simulink library "ipc"  (Simulink 8.1)
settings: Solver=ode1  StartTime=0.0  StopTime=Inf  FixedStep=0.001  RelTol=1e-3
PostLoadFcn:
  | , if any(exist('dsrtsu_mdlpostloadfcn', 'file') == [2, 3, 6]), try dsrtsu_mdlpostloadfcn('Execute', bdroot); catch fprintf('Error in PostLoadFcn (dsrtsu_mdlpostloadfcn) for model "%s":\n %s\n', bdroot, lasterr); end, end,
undefined symbols (not defined in the file or in its folder): KIFO_OffsetToBumper_m, KIFO_TTCDefault_s
libraries: hcu_lib x2, ltc x1
settings Model: DSRTSU_INTERNAL_RTI_VER=450  DSRTSU_INTERNAL_RTI_TYPE=rti1401  RTICANMMDATA=struct('GeneralSetupData',struct('modelroot',['D:\ELN150201\Phase3\branches\Pedestrians complete local\AdasDragon\software\sw_development\arch\app\ifo'],'generalsettings',struct('filesettings',struct('destfolder',struct('Name','RTICANMM_FILES','Check',1),'buildfolder',struct('Name','.','Check',1),'AbsDestfolder',struct('Name',['D:\ELN150201\Phase3\branches\Pedestrians complete local\AdasDragon\software\sw_development\arch\app\ifo\RTICANMM_FILES']),'AbsBuildfolder',struct('Name',['D:\ELN150201\Phase3\branches\Pedestrians complete local\AdasDragon\software\sw_development\arch\app\ifo']))),'options',struct('addpaths',1,'rmpaths',1,'addtrcexclusion',logical(1),'cannavigator',struct('checkmonitoring',0),'show_usrtrc',0,'use_usrtrc',0),'advanced',struct('options',[1 1 1 1 1 1 1 1 1 1 1 1 1 1 1 1 1 1 1 1 1 1 1 1 1 1 1 1 1 1 1 1 1 1 1 1 1 1 1 1 1 1 1 1 1 1 1 1 1 1 1 1 1 1 1 1 1 1 1 1 1 1 1 1 1 1 1 1 1 1 1 1 1 1 1 1 1 1 1 1 1 1 1 1 1 1 1 1 1 1 1 1 1 1 1 1 1 1 1 1]),'MPSetup',{{}},'modelname','ipc','block','ipc'))  DSRTSU_INTERNAL_RTIFPGA=40  Creator=tescamilla  LastModifiedBy=AT015555

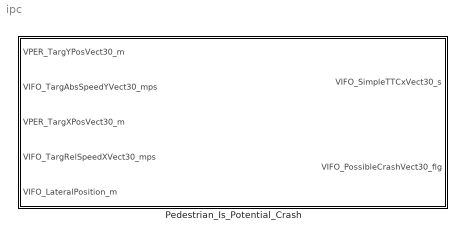
== system ipc ==
  Pedestrian_Is_Potential_Crash : Subsystem

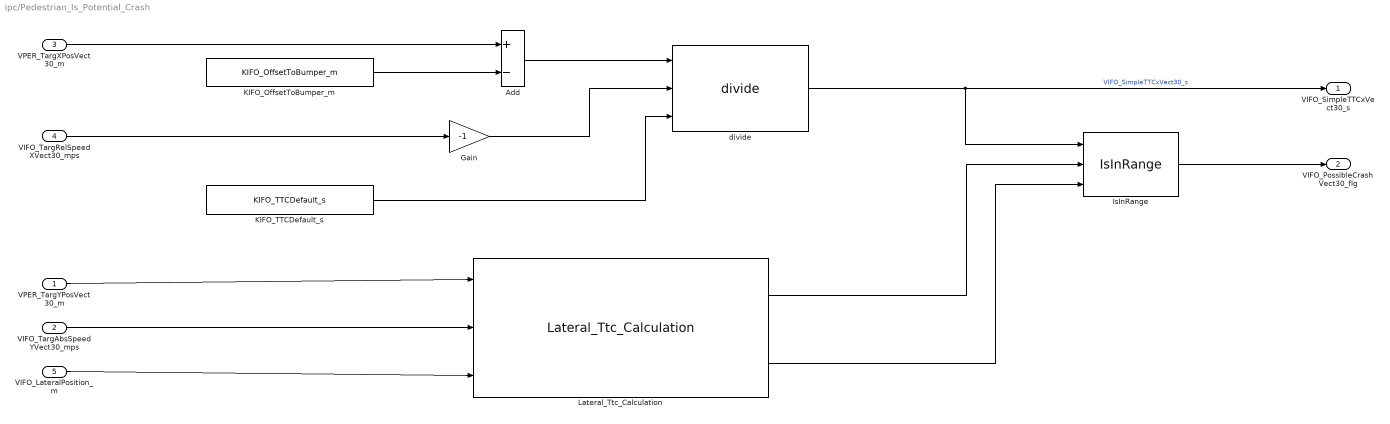
== system ipc/Pedestrian_Is_Potential_Crash ==
  VPER_TargYPosVect30_m : Inport
  VIFO_TargAbsSpeedYVect30_mps : Inport  Port=2
  VPER_TargXPosVect30_m : Inport  Port=3
  VIFO_TargRelSpeedXVect30_mps : Inport  Port=4
  VIFO_LateralPosition_m : Inport  Port=5
  Add : Sum  Inputs=+-
  Gain : Gain  Gain=-1
  IsInRange : hcu_lib/IsInRange  SystemSampleTime=-1
  KIFO_OffsetToBumper_m : Constant  Value=KIFO_OffsetToBumper_m
  KIFO_TTCDefault_s : Constant  Value=KIFO_TTCDefault_s
  Lateral_Ttc_Calculation : ltc/Lateral_Ttc_Calculation
  divide : hcu_lib/divide
  VIFO_SimpleTTCxVect30_s : Outport
  VIFO_PossibleCrashVect30_flg : Outport  Port=2
  wires:
  VPER_TargYPosVect30_m/1 -> Lateral_Ttc_Calculation/1
  VPER_TargXPosVect30_m/1 -> Add/1
  KIFO_OffsetToBumper_m/1 -> Add/2
  VIFO_TargRelSpeedXVect30_mps/1 -> Gain/1
  Add/1 -> divide/1
  Gain/1 -> divide/2
  KIFO_TTCDefault_s/1 -> divide/3
  VIFO_TargAbsSpeedYVect30_mps/1 -> Lateral_Ttc_Calculation/2
  Lateral_Ttc_Calculation/1 -> IsInRange/2
  divide/1 -> IsInRange/1, VIFO_SimpleTTCxVect30_s/1  "VIFO_SimpleTTCxVect30_s"
  Lateral_Ttc_Calculation/2 -> IsInRange/3
  IsInRange/1 -> VIFO_PossibleCrashVect30_flg/1
  VIFO_LateralPosition_m/1 -> Lateral_Ttc_Calculation/3
